simulink model "modules_intentions"  (R2017a)
settings: Solver=ode4  StartTime=0.0  StopTime=time_stop  FixedStep=time_step  RelTol=1e-3
undefined symbols (not defined in the file or in its folder): beta, Delta_guidance, Delta_matrix, eta_initial, initial_desired_psi_vector, initial_desired_u_vector, initial_next_waypoint_indexes, initial_obstacle_ship_states, initial_obstacle_ship_states_dot, initial_reference_psi_vector, initial_reference_u_vector, initial_SBMPC_desired_psi_vector, initial_SBMPC_desired_u_vector, initial_SBMPC_next_waypoint_indexes, initial_SBMPC_obstacle_ship_states, initial_SBMPC_obstacle_ship_states_dot, initial_SBMPC_reference_psi_vector, initial_SBMPC_reference_u_vector, initial_SBMPC_x_d_psi_matrix, initial_SBMPC_x_d_u_matrix, initial_state, initial_x_d_psi_matrix, initial_x_d_u_matrix, K_sway, K_yaw, Kp_feedback_linearization, kp_heading, Nmax, nu_initial, num_obs_ship_waypoints, num_prediction_time_steps, number_of_control_behaviors, number_of_obstacle_ships, number_of_SBMPC_obstacle_ships, obs_speed_between_waypoints, obstacle_waypoint_matrix, Omega_matrix, own_ship_reference_psi_init, own_ship_reference_speed, psi, Psi_init, radius_of_acceptance, SBMPC_obs_speed_between_waypoints, SBMPC_obstacle_waypoint_matrix, seconds_between_prediction, state_vector_init, T, T_k_surge, T_k_sway, T_k_yaw, T_s, T_waypoints, time_step, tsamp, U, U_init, V_init, waypoints_obstacle_ships, waypoints_own_ship, Xmax ... (+1)
(part 3 of 6)

== system modules_intentions/SBMPC obstacle ships/SBMPC using intentions /SBMPC obstacles: own-ship trajectory prediction ==
  note: each row = time step in prediction horizion
      | each column = a different control scenario
  note: each row = time step in prediction horizion
      | each column = a different control scenario
  note: each row = time step in prediction horizion
      | each column = a different control scenario
  note: each row = time step in prediction horizion
      | each column = a different control scenario
  note: each row = time step in prediction horizion
      | each column = a different control scenario
  t_0 : Inport
  SBMPC_obs_waypoints_matrix : Inport  Port=2
  "SBMPC_obs_eta_initial " : Inport  Port=3
  SBMPC_obs_nu_initial : Inport  Port=4
  SBMPC_obs_next_waypoint_index : Inport  Port=5
  Own ship trajectory prediction : MATLAB Function  TreatAsAtomicUnit=on
  To Workspace1 : ToWorkspace  Commented=on  VariableName=SBMPC_own_ship_x_predicted  SaveFormat=Structure With Time  SampleTime=tsamp
  To Workspace3 : ToWorkspace  Commented=on  VariableName=SBMPC_own_ship_y_predicted  SaveFormat=Structure With Time  SampleTime=tsamp
  To Workspace4 : ToWorkspace  Commented=on  VariableName=SBMPC_own_ship_heading_predicted  SaveFormat=Structure With Time  SampleTime=tsamp
  To Workspace5 : ToWorkspace  Commented=on  VariableName=SBMPC_own_ship_u_predicted  SaveFormat=Structure With Time  SampleTime=tsamp
  To Workspace6 : ToWorkspace  Commented=on  VariableName=SBMPC_own_ship_v_predicted  SaveFormat=Structure With Time  SampleTime=tsamp
  SBMPC_obs_own_ship_x_predicted : Outport  SampleTime=time_step
  SBMPC_obs_own_ship_y_predicted : Outport  Port=2  SampleTime=time_step
  SBMPC_obs_own_ship_heading_predicted : Outport  Port=3  SampleTime=time_step
  SBMPC_obs_own_ship_u_predicted : Outport  Port=4  SampleTime=time_step
  "SBMPC_obs_own_ship_v_predicted " : Outport  Port=5  SampleTime=time_step
  wires:
  SBMPC_obs_waypoints_matrix/1 -> Own ship trajectory prediction/4(waypoints_matrix)
  SBMPC_obs_nu_initial/1 -> Own ship trajectory prediction/3(nu_initial)
  "SBMPC_obs_eta_initial "/1 -> Own ship trajectory prediction/2(eta_initial)
  SBMPC_obs_next_waypoint_index/1 -> Own ship trajectory prediction/5(next_waypoint_index)
  t_0/1 -> Own ship trajectory prediction/1(t_0)
  Own ship trajectory prediction/1(own_ship_x_predicted) -> SBMPC_obs_own_ship_x_predicted/1, To Workspace1/1
  Own ship trajectory prediction/2(own_ship_y_predicted) -> SBMPC_obs_own_ship_y_predicted/1, To Workspace3/1
  Own ship trajectory prediction/3(own_ship_heading_predicted) -> To Workspace4/1, SBMPC_obs_own_ship_heading_predicted/1
  Own ship trajectory prediction/4(own_ship_u_predicted) -> SBMPC_obs_own_ship_u_predicted/1, To Workspace5/1
  Own ship trajectory prediction/5(own_ship_v_predicted) -> "SBMPC_obs_own_ship_v_predicted "/1, To Workspace6/1

== matlab function modules_intentions/Own-ship/Own-ship PSV/PSV/PSV model ==
  data: Pr input; psi_ca input; desired_nu input; state output; desired_psi input; time_step parameter; eta_initial parameter; nu_initial parameter; tau output; Kp_feedback_linearization parameter; kp_heading parameter; Xmax parameter; Ymax parameter; Nmax parameter; K_sway parameter; K_yaw parameter; T_k_surge parameter; T_k_sway parameter; T_k_yaw parameter
function [state, tau]   = PSV(Pr, psi_ca, desired_nu, desired_psi, time_step, eta_initial, nu_initial, Kp_feedback_linearization, kp_heading, Xmax, Ymax, Nmax, K_sway, K_yaw, T_k_surge, T_k_sway, T_k_yaw)  
    desired_u = desired_nu(1);
    desired_v = desired_nu(2);
    desired_r = desired_nu(3);

    persistent psv_vessel; %Persistent variables are local to the function in which they are declared, yet their values are retained in memory between calls to the function.
    
    if (isempty(psv_vessel))
        psvParameters = coder.load('PSVparameters');
        psvModelParameters = psvParameters.model_config;
        psv_vessel = PSVvessel_class(psvModelParameters, eta_initial, nu_initial, time_step, desired_psi, desired_nu, Kp_feedback_linearization, kp_heading, Xmax, Ymax, Nmax, K_sway, K_yaw, T_k_surge, T_k_sway, T_k_yaw);
    end
    
    desired_psi = desired_psi + psi_ca;
    desired_nu(1) = desired_nu(1)*Pr;

    
    [psv_vessel, tau] = psv_vessel.update_states(desired_psi, desired_nu);           
    state = psv_vessel.state;   
end

== matlab function modules_intentions/Own-ship/reference model psi/own ship reference model psi ==
  data: reference_psi input; x_d_new output; Omega_matrix parameter; time_step parameter; eta_initial parameter
function x_d_new = ownShipReferenceModelPsi(reference_psi, Omega_matrix, time_step, eta_initial)

persistent x_d %%[eta; eat_dot; eta_dotdot] = [x,y,psi, x_dot, y_dot, psi_dot, x_ddot, y_ddot, psi_ddot]

if isempty(x_d)
    x_d = [eta_initial(1);eta_initial(2);eta_initial(3);0;0;0;0;0;0];
end

x_d = referenceModelPsi(x_d, reference_psi, Omega_matrix, time_step);
x_d_new = x_d;
end

== matlab function modules_intentions/Own-ship/SBMPC USING INTENTIONS /Calculate control behaviors/Compute hazard ==
  settings: updateMethod=DISCRETE  sampleTime=time_step
  data: obstacle_ships_u input size=[num_prediction_time_steps, total_number_of_obstacle_ships]; obstacle_ships_v input size=[num_prediction_time_steps, total_number_of_obstacle_ships]; obstacle_ships_psi input size=[num_prediction_time_steps, total_number_of_obstacle_ships]; t_0 input; own_ship_x_predicted input size=[num_prediction_time_steps, number_of_control_behaviors]; own_ship_y_predicted input size=[num_prediction_time_steps, number_of_control_behaviors]; own_ship_u_predicted input size=[num_prediction_time_steps, number_of_control_behaviors]; own_ship_v_predicted input size=[num_prediction_time_steps, number_of_control_behaviors]; own_ship_heading_predicted input size=[num_prediction_time_steps, number_of_control_behaviors]; CLOSE output size=[number_of_control_behaviors, total_number_of_obstacle_ships, num_prediction_time_steps]; d_0 output size=[number_of_control_behaviors, total_number_of_obstacle_ships, num_prediction_time_steps]; obstacle_ships_x_predicted input size=[num_prediction_time_steps, total_number_of_obstacle_ships]; obstacle_ships_y_predicted input size=[num_prediction_time_steps, total_number_of_obstacle_ships]; OVERTAKEN output size=[number_of_control_behaviors, total_number_of_obstacle_ships, num_prediction_time_steps]; STARBOARD output size=[number_of_control_behaviors, total_number_of_obstacle_ships, num_prediction_time_steps]; chosen_HEAD_ON_out output; CROSSED output size=[number_of_control_behaviors, total_number_of_obstacle_ships, num_prediction_time_steps]; mu output size=[number_of_control_behaviors, total_number_of_obstacle_ships, num_prediction_time_steps]; num_prediction_time_steps parameter; heading_angle_offset_commands parameter; propulsion_commands parameter; total_number_of_obstacle_ships parameter; seconds_between_prediction parameter; d_cl parameter; phi_head_on parameter; phi_crossed parameter; phi_overtaken parameter; phi_ahead parameter; K_coll parameter; C output size=number_of_control_behaviors, total_number_of_obstacle_ships, num_prediction_time_steps; R output size=number_of_control_behaviors, total_number_of_obstacle_ships, num_prediction_time_steps; q parameter; p parameter; d_safe parameter; k_boundary parameter; k_circle parameter; k_Pr parameter; k_psi_port parameter; k_psi_starboard parameter; Delta_Pr parameter; vessel_length parameter; circle_obstacle_parameters parameter; boundary_obstacles_parameters parameter; k_Delta_psi_port parameter; k_Delta_psi_starboard parameter; kappa parameter; f output size=[1,number_of_control_behaviors]; g output size=[1,number_of_control_behaviors]; hazard output size=[1,number_of_control_behaviors]; rad2deg parameter; num_boundary_obstacles parameter; num_circle_obstacles parameter; chosen_C_out output; chosen_P_out output; chosen_FC_out output; chosen_R_out output; chosen_scaled_mu_out output; T_s parameter; chosen_Pr_out output; chosen_psi_ca_out output; C_worst output; R_worst output; scaled_mu_worst output; Pr_worst output; psi_ca_worst output; f_worst_out output; g_worst_out output; smallest_hazard_out output; largest_hazard_out output; f_out output; g_out output; r parameter; R_vector_out output size=[number_of_control_behaviors, total_number_of_obstacle_ships, num_prediction_time_steps]; circle_safety_margin parameter; p_boundary parameter; p_circle parameter; q_circle parameter; q_boundary parameter; boundary_margin parameter; k_role parameter; L_role parameter; ROLE_realtive_to_own_ship_module parameter; L_FC parameter; k_FC parameter; number_of_control_behaviors parameter; HEAD_ON_realtive_to_own_ship_module parameter; chosen_scenario_index_out output; t_detect_out output size=[1, total_number_of_obstacle_ships]; changing_obs parameter; number_of_obstacle_ships parameter; L_C parameter
 function [CLOSE, d_0, OVERTAKEN, STARBOARD, chosen_HEAD_ON_out, CROSSED,mu, C, R, f, g, hazard, chosen_C_out, chosen_P_out, chosen_FC_out, chosen_R_out, chosen_scaled_mu_out, chosen_Pr_out, chosen_psi_ca_out, C_worst, R_worst, scaled_mu_worst, Pr_worst, psi_ca_worst, f_worst_out, g_worst_out, smallest_hazard_out, largest_hazard_out, f_out, g_out, R_vector_out, chosen_scenario_index_out, t_detect_out]                         = computeTotalHazard(obstacle_ships_u, obstacle_ships_v, obstacle_ships_psi, t_0,own_ship_x_predicted, own_ship_y_predicted,own_ship_u_predicted,own_ship_v_predicted, own_ship_heading_predicted, obstacle_ships_x_predicted, obstacle_ships_y_predicted, num_prediction_time_steps, heading_angle_offset_commands, propulsion_commands, total_number_of_obstacle_ships, seconds_between_prediction, d_cl,phi_head_on, phi_crossed, phi_overtaken,phi_ahead,K_coll, q, p, d_safe,k_boundary, k_circle, k_Pr, k_psi_port, k_psi_starboard, Delta_Pr, vessel_length, circle_obstacle_parameters, boundary_obstacles_parameters, k_Delta_psi_port, k_Delta_psi_starboard,kappa, rad2deg, num_boundary_obstacles, num_circle_obstacles, T_s, r,  circle_safety_margin, p_boundary, p_circle, q_circle, q_boundary, boundary_margin, k_role, L_role, ROLE_realtive_to_own_ship_module, L_FC, k_FC, number_of_control_behaviors, HEAD_ON_realtive_to_own_ship_module, changing_obs, number_of_obstacle_ships, L_C)
    persistent chosen_C;
    persistent chosen_scenario_index;
    persistent chosen_R;
    persistent chosen_scaled_mu;
    persistent chosen_P_role;
    persistent chosen_FC;
    persistent chosen_HEAD_ON;
    persistent chosen_Pr;
    persistent chosen_psi_ca;
    persistent chosen_Pr_worst;
    persistent chosen_psi_ca_worst;
    persistent f_worst;
    persistent g_worst;
    persistent f_chosen;
    persistent g_chosen;
    persistent smallest_hazard;
    persistent largest_hazard;
    persistent scenario_index_with_min_hazard;
    persistent scenario_index_with_max_hazard;
    persistent t_detect;
    persistent t_detect_update;
    
    if (isempty(chosen_C))
        chosen_C = zeros(1,number_of_control_behaviors);%chosen_C_init;
        chosen_scenario_index = 0;
        chosen_R = zeros(1,number_of_control_behaviors);%chosen_R_init;
        chosen_scaled_mu = zeros(1,number_of_control_behaviors);%chosen_scaled_mu_init; 
        chosen_P_role = zeros(1,number_of_control_behaviors);%chosen_P_role_init;
        chosen_FC     = zeros(1,number_of_control_behaviors);
        chosen_HEAD_ON = zeros(1,number_of_control_behaviors);
        chosen_Pr = 1;
        chosen_psi_ca = 0;
        chosen_Pr_worst = 0;
        chosen_psi_ca_worst = 0;
        f_worst = 0;
        g_worst = 0;
        f_chosen = 0;
        g_chosen = 0;
        smallest_hazard = 0;
        largest_hazard = 0;
        scenario_index_with_min_hazard = -1;
        scenario_index_with_max_hazard = -1;
        t_detect = ones(1, total_number_of_obstacle_ships)*(-1);
        t_detect_update = ones(1, total_number_of_obstacle_ships);
        
    end

    CLOSE     = zeros(number_of_control_behaviors, total_number_of_obstacle_ships, num_prediction_time_steps);%CLOSE_init;         %3D matrix, 1. dim: scenario, 2. dim: obstacle, 3. dim: prediction horizon time step.
    OVERTAKEN = zeros(number_of_control_behaviors, total_number_of_obstacle_ships, num_prediction_time_steps);%OVERTAKEN_init; %3D matrix, 1. dim: scenario, 2. dim: obstacle, 3. dim: prediction horizon time step.
    STARBOARD = zeros(number_of_control_behaviors, total_number_of_obstacle_ships, num_prediction_time_steps);%STARBOARD_init; %3D matrix, 1. dim: scenario, 2. dim: obstacle, 3. dim: prediction horizon time step.
    HEAD_ON   = zeros(number_of_control_behaviors, total_number_of_obstacle_ships, num_prediction_time_steps);%HEAD_ON_init;     %3D matrix, 1. dim: scenario, 2. dim: obstacle, 3. dim: prediction horizon time step.
    CROSSED   = zeros(number_of_control_behaviors, total_number_of_obstacle_ships, num_prediction_time_steps);%CROSSED_init;     %3D matrix, 1. dim: scenario, 2. dim: obstacle, 3. dim: prediction horizon time step.
    mu        = zeros(number_of_control_behaviors, total_number_of_obstacle_ships, num_prediction_time_steps);%mu_init;               %3D matrix, 1. dim: scenario, 2. dim: obstacle, 3. dim: prediction horizon time step.
    scaled_mu = zeros(number_of_control_behaviors, total_number_of_obstacle_ships, num_prediction_time_steps);%scaled_mu_init; %3D matrix, 1. dim: scenario, 2. dim: obstacle, 3. dim: prediction horizon time step.
    d_0       = zeros(number_of_control_behaviors, total_number_of_obstacle_ships, num_prediction_time_steps);%d_0_init;             %3D matrix. distance between own ship and obstacle ship i at time t in scenario k. 1. dim: scenario, 2. dim: obstacle, 3. dim: prediction horizon time step
    f         = zeros(1,number_of_control_behaviors);%f_init;                 %vector.
    g         = zeros(1,number_of_control_behaviors);%g_init;                 %vector
    
    
    if (num_circle_obstacles > 0)
        g_circle_init  = zeros(number_of_control_behaviors, num_circle_obstacles, num_prediction_time_steps);
    else
        g_circle_init = 0;
    end    
    if (num_boundary_obstacles > 0)
        g_boundary_init = zeros(number_of_control_behaviors, num_boundary_obstacles, num_prediction_time_steps);
    else
        g_boundary_init = 0;
    end 
    g_circle  = g_circle_init;       %3D matrix. 1. dim = scneario, 2. dim = circle obstacle index, 3. dim = prediction horizon time step.
    g_boundary = g_boundary_init;   %3D matrix. 1. dim = scneario, 2. dim = circle obstacle index, 3. dim = prediction horizon time step.
    C = zeros(number_of_control_behaviors, total_number_of_obstacle_ships, num_prediction_time_steps);%C_init; %cost of collision. 3D matrix, 1. dim: scenario, 2. dim: obstacle, 3. dim: prediction horizon time step.
    R = zeros(number_of_control_behaviors, total_number_of_obstacle_ships, num_prediction_time_steps);%R_init; %Risk of collision. 3D matrix, 1. dim: scenario, 2. dim: obstacle, 3. dim: prediction horizon time step.
    hazard = zeros(1,number_of_control_behaviors);%hazard_init;
    P_role = zeros(number_of_control_behaviors, total_number_of_obstacle_ships, num_prediction_time_steps);%P_role_init;
    FC = zeros(number_of_control_behaviors, total_number_of_obstacle_ships, num_prediction_time_steps);%FC_init;
    
     
    Pr_last = chosen_Pr;     %the Pr corresponding to the previously calculated lowest hazard.
    psi_ca_last = chosen_psi_ca;    
    if (t_0 == 0)
        Pr_last = 1;
        psi_ca_last = 0;
    end
    
    if (mod(t_0, seconds_between_prediction) == 0) %only compute every "seconds_between_prediction" second.
        scenario_index = 0;
        for Pr = propulsion_commands
            for psi_ca = heading_angle_offset_commands 
                scenario_index = scenario_index + 1;                      
                prediction_time = 0;
                for t=1:num_prediction_time_steps   
                    prediction_time = t_0 + t*T_s;

                    %%%% Penalty for static obstacles   
                    if (num_circle_obstacles > 0)
                        circle_obs_counter = 0;
                        for circle_obstacle = circle_obstacle_parameters.'         %in each iteration, circle_obstacle is column vector with [radius; center_x; center_y]
                            circle_obs_counter = circle_obs_counter + 1;
                            radius    = circle_obstacle(1);
                            center_x  = circle_obstacle(2);
                            center_y  = circle_obstacle(3);
                            crossing_with_circle = SBMPC_isCollisionWithCircleObstacle(own_ship_x_predicted(t,scenario_index), own_ship_y_predicted(t,scenario_index), vessel_length, own_ship_heading_predicted(t,scenario_index), center_x, center_y, radius, circle_safety_margin);                       
                            vessel_bow_x = own_ship_x_predicted(t,scenario_index) + cos(own_ship_heading_predicted(t,scenario_index))*(vessel_length/2);
                            vessel_bow_y = own_ship_y_predicted(t,scenario_index) + sin(own_ship_heading_predicted(t,scenario_index))*(vessel_length/2);
                            distance_bow_to_circle_center = sqrt( (center_x - vessel_bow_x)^2 + (center_y - vessel_bow_y)^2 );
                            g_circle(scenario_index, circle_obs_counter, t) = (crossing_with_circle+1)*k_circle*(1/(prediction_time - t_0)^p_circle)*((radius+L_C)/ distance_bow_to_circle_center)^q_circle;%*(psi_ca*rad2deg)     * (1/distance_bow_to_circle_center)                   
                       end % end for
                    end % end if                        

                    if (num_boundary_obstacles > 0)
                        boundary_obs_counter = 0;
                        for boundary_obstacle = boundary_obstacles_parameters.'
                            boundary_obs_counter = boundary_obs_counter + 1;
                            boundary_start_x = boundary_obstacle(1);
                            boundary_start_y = boundary_obstacle(2);
                            boundary_end_x   = boundary_obstacle(3);
                            boundary_end_y   = boundary_obstacle(4);  
                            vessel_bow_x = own_ship_x_predicted(t,scenario_index) + cos(own_ship_heading_predicted(t,scenario_index))*(vessel_length/2);
                            vessel_bow_y = own_ship_y_predicted(t,scenario_index) + sin(own_ship_heading_predicted(t,scenario_index))*(vessel_length/2);
                            distance_bow_to_line = dist_from_bow_to_line( vessel_bow_x, vessel_bow_y, boundary_start_x, boundary_start_y, boundary_end_x, boundary_end_y ); % from http://paulbourke.net/geometry/pointlineplane/
                            crossing_with_boundary = SBMPC_isCollisionWithBoundaryObstacle(own_ship_x_predicted(t,scenario_index), own_ship_y_predicted(t,scenario_index), vessel_length, own_ship_heading_predicted(t,scenario_index), boundary_start_x, boundary_start_y, boundary_end_x, boundary_end_y);
                            g_boundary(scenario_index, boundary_obs_counter, t) = (crossing_with_boundary+1)*k_boundary*( 1 / (prediction_time - t_0)^p_boundary )*((boundary_margin)/(distance_bow_to_line))^q_boundary;  %from wiki https://en.wikipedia.org/wiki/Distance_from_a_point_to_a_line
                        end % end for
                    end % end if

                    for obstacle_ship_index = 1:total_number_of_obstacle_ships
                        obstacle_ship_speed = sqrt(obstacle_ships_u(t,obstacle_ship_index)^2 + obstacle_ships_v(t,obstacle_ship_index)^2);
                        own_ship_speed = sqrt(own_ship_u_predicted(t,scenario_index)^2 + own_ship_v_predicted(t,scenario_index)^2);
                        own_ship_u_NED = own_ship_speed*cos(own_ship_heading_predicted(t,scenario_index));
                        own_ship_v_NED = own_ship_speed*sin(own_ship_heading_predicted(t,scenario_index));
                        obstacle_ship_u_NED = obstacle_ship_speed*cos(obstacle_ships_psi(t,obstacle_ship_index));  
                        obstacle_ship_v_NED = obstacle_ship_speed*sin(obstacle_ships_psi(t,obstacle_ship_index));               
                        V_0 = [own_ship_u_NED,own_ship_v_NED];
                        V_i = [obstacle_ship_u_NED, obstacle_ship_v_NED];       
                                                
                        d_0(scenario_index, obstacle_ship_index, t) = sqrt((own_ship_x_predicted(t,scenario_index) - obstacle_ships_x_predicted(t,obstacle_ship_index))^2 ...
                                                                        +  (own_ship_y_predicted(t,scenario_index) - obstacle_ships_y_predicted(t,obstacle_ship_index))^2); 
                                                                    
                        if ( obstacle_ship_index <= number_of_obstacle_ships)   
                            if (changing_obs(obstacle_ship_index) == 1) %if it is a normal obs ship AND this normal obs ship is changing her waypoints midway in scenario
                                t_detect(obstacle_ship_index) = 1;
                                t_detect_update(obstacle_ship_index) = false;
                            elseif(changing_obs(obstacle_ship_index) == 0 && d_0(scenario_index, obstacle_ship_index, t) <= d_safe(obstacle_ship_index) && t_detect_update(obstacle_ship_index) == true)
                                t_detect(obstacle_ship_index) = t_0;
                                t_detect_update(obstacle_ship_index) = false;
                            end
                        elseif(obstacle_ship_index >number_of_obstacle_ships ) 
                            if (d_0(scenario_index, obstacle_ship_index, t) <= d_safe(obstacle_ship_index) && t_detect_update(obstacle_ship_index) == true)
                                t_detect(obstacle_ship_index) = t_0;
                                t_detect_update(obstacle_ship_index) = false;    
                            end
                        end
                                                                    
                        %%%% CLOSE
                                                                    
                        if (d_0(scenario_index, obstacle_ship_index, t) <= d_cl(obstacle_ship_index))
                            CLOSE(scenario_index, obstacle_ship_index, t) = 1;
                        else
                            CLOSE(scenario_index, obstacle_ship_index, t) = 0;
                        end % end if

                        %%%% OVERTAKEN                  
                        %equation 5 in johansen
                        epsilon = 1;
                        if (CLOSE(scenario_index, obstacle_ship_index, t) == 1 && obstacle_ship_speed > own_ship_speed + epsilon && dot(V_0, V_i) > cos(phi_overtaken)*norm(V_0)*norm(V_i))
                            OVERTAKEN(scenario_index, obstacle_ship_index, t) = 1;
                        else
                            OVERTAKEN(scenario_index, obstacle_ship_index, t) = 0;
                        end % end if

                        %%%% STARBOARD
                        L = [ obstacle_ships_x_predicted(t,obstacle_ship_index) - own_ship_x_predicted(t,scenario_index) , obstacle_ships_y_predicted(t,obstacle_ship_index) - own_ship_y_predicted(t,scenario_index) ];
                        L_unit_vector = L/norm(L);
                        L_angle = atan2(  (obstacle_ships_y_predicted(t,obstacle_ship_index) - own_ship_y_predicted(t,scenario_index)) , (obstacle_ships_x_predicted(t,obstacle_ship_index) - own_ship_x_predicted(t,scenario_index))  );

                        if (L_angle > own_ship_heading_predicted(t,scenario_index))
                            STARBOARD(scenario_index, obstacle_ship_index, t) = 1;
                        else
                            STARBOARD(scenario_index, obstacle_ship_index, t) = 0;
                        end
                        %rad2deg = 180/pi;
                        %L_angle_deg = L_angle*rad2deg;
                        %L_angle_deg_converted_to_positive =  mod((L_angle_deg + 360), 360);
                        %L_angle_mapped = L_angle_deg_converted_to_positive*deg2rad;  %map negative angles to positive angles.

                        %%%% HEAD_ON
                        head_on_condition = false;
                        if ( dot(V_0, V_i) < -cos(phi_head_on)*norm(V_0)*norm(V_i) && dot(V_0, L_unit_vector) > cos(phi_ahead)*norm(V_0) ) 
                            head_on_condition = true ; %equation 6-7 in johansen paper 
                        end% end if

                        if (CLOSE(scenario_index, obstacle_ship_index, t) == 1 && norm(V_i) ~= 0 && head_on_condition == true )
                            HEAD_ON(scenario_index, obstacle_ship_index, t) = 1;
                        else
                            HEAD_ON(scenario_index, obstacle_ship_index, t) = 0;
                        end % end if

                        %%%% CROSSED                                              
                        if (CLOSE(scenario_index, obstacle_ship_index, t) == 1 && dot(V_0, V_i) < cos(phi_crossed)*norm(V_0)*norm(V_i))
                            CROSSED(scenario_index, obstacle_ship_index, t) = 1;
                        else
                            CROSSED(scenario_index, obstacle_ship_index, t) = 0;
                        end % end if
                                                
                        %%%% RULE14    
                        if (CLOSE(scenario_index, obstacle_ship_index, t) == 1 && STARBOARD(scenario_index, obstacle_ship_index, t) == 1 && HEAD_ON(scenario_index, obstacle_ship_index, t) == 1 )
                            RULE14 = true;
                        else
                            RULE14 = false;
                        end % end if

                        %%%% RULE15   
                        if (CLOSE(scenario_index, obstacle_ship_index, t) == 1 && STARBOARD(scenario_index, obstacle_ship_index, t) == 1 && CROSSED(scenario_index, obstacle_ship_index, t) == 1 && OVERTAKEN(scenario_index, obstacle_ship_index, t)== 0 )
                            RULE15 = true;
                        else
                             RULE15 = false;
                        end % end if

                        %%%% mu
                        if (RULE14 || RULE15)
                            mu(scenario_index, obstacle_ship_index, t) =  1;
                        else
                            mu(scenario_index, obstacle_ship_index, t) = 0;
                        end % end if                         
                        scaled_mu(scenario_index, obstacle_ship_index, t) = kappa(obstacle_ship_index)*mu(scenario_index, obstacle_ship_index, t);
                        
                        
                        %%%% Role variable 
                        if (CLOSE(scenario_index, obstacle_ship_index, t) == 1 && d_0(scenario_index, obstacle_ship_index, t) >= L_role)
                            HEAD_ON_intention_value = HEAD_ON_realtive_to_own_ship_module(obstacle_ship_index);
                            P_role(scenario_index, obstacle_ship_index, t) = ROLE_realtive_to_own_ship_module(obstacle_ship_index)*k_role*(1-HEAD_ON_intention_value)*(sqrt(abs(psi_ca*rad2deg)) + 1 - Pr);        
                        else
                            P_role(scenario_index, obstacle_ship_index, t) = 0;
                        end % end if
                        
                        
                                                                 
                        %%%% Cost of collision
                        C(scenario_index, obstacle_ship_index, t) = K_coll(obstacle_ship_index)*norm(V_0 - V_i)^2;
                        
                        %%%% Risk of collision    
                        
                        if (d_0(scenario_index, obstacle_ship_index, t) <= L_FC)
                            FC(scenario_index, obstacle_ship_index, t) = 1;
                        else
                            FC(scenario_index, obstacle_ship_index, t) = 0;
                        end % end if
                        
                        
                        if (d_0(scenario_index, obstacle_ship_index, t) <= d_safe(obstacle_ship_index) && d_0(scenario_index, obstacle_ship_index, t) >= 20)                          
                            R(scenario_index, obstacle_ship_index, t)  = (1 / (abs(prediction_time - t_0)^p))*( r*( d_safe(obstacle_ship_index) / d_0(scenario_index, obstacle_ship_index, t) )^q  + k_FC*FC(scenario_index, obstacle_ship_index, t)   ) ;
                            if ( R(scenario_index, obstacle_ship_index, t) >= 20000)
                                R(scenario_index, obstacle_ship_index, t) = 20000;  %saturate
                            end
                        else
                            R(scenario_index, obstacle_ship_index, t) = 0;
                        end % end if        
                        
                    end % end for - num obs ships            
                end % end for - time steps                                        
            end % end for - psi_ca
        end % end for - Pr     
        
        scenario_index = 0;
        for Pr = propulsion_commands
            for psi_ca = heading_angle_offset_commands 
                scenario_index = scenario_index + 1;
                sum_matrix = C(scenario_index,:,:).*R(scenario_index,:,:) + scaled_mu(scenario_index,:,:) + P_role(scenario_index,:,:);   %sum matrix: 1. dim = control behavior, 2. dim = obstacle, 3. dim = prediction horizon time step.
                %assert (size(sum_matrix) == [1, total_number_of_obstacle_ships, num_prediction_time_steps]);
                sum_matrix = reshape(sum_matrix, total_number_of_obstacle_ships, num_prediction_time_steps);
                [best_value,idx] = max(sum_matrix(:));
                [best_obstacle_ship_index,best_timestep] = ind2sub(size(sum_matrix),idx);
                  
                  %ALTERNATIVE WAY TO FIND MAXIMUMS
%                 max_sum = -1;
%                 i_ = 0;
%                 t_ = 0;
%                 
%                 for i = 1:total_number_of_obstacle_ships
%                     for t = 1:num_prediction_time_steps
%                         sum = C(scenario_index, i, t)*R(scenario_index, i, t) + scaled_mu(scenario_index, i, t) + P_role(scenario_index, i, t);
%                         if (sum > max_sum)
%                             max_sum = sum;
%                             i_ = i;
%                             t_ = t;
%                         end % end if
%                     end % end for
%                 end % end for%                 
%                 assert (best_value == max_sum);                            
                
                if ( psi_ca < 0)
                    k_psi = k_psi_port;  
                    Delta_psi = k_Delta_psi_port*(abs(psi_ca*rad2deg - psi_ca_last*rad2deg));
                else
                    k_psi = k_psi_starboard;
                    Delta_psi = k_Delta_psi_starboard*(abs(psi_ca*rad2deg - psi_ca_last*rad2deg));
                end % end if                
                
                f(scenario_index) = k_Pr*(1-Pr) + k_psi*(abs(psi_ca*rad2deg)) + Delta_Pr*abs(Pr - Pr_last) + Delta_psi ;                                 
                
                g_circle_scenario = 0;
                if (num_circle_obstacles > 0)
                    g_circle_scenario_values = g_circle(scenario_index, :, :);
                    g_circle_scenario = max(g_circle_scenario_values(:));
                end % end if                
                g_boundary_scenario = 0;
                if (num_boundary_obstacles > 0)
                    g_boundary_scenario_values = g_boundary(scenario_index, :, :);
                    g_boundary_scenario = max(g_boundary_scenario_values(:));
                end % end if                
                g(scenario_index) = g_circle_scenario + g_boundary_scenario;
                
                hazard(scenario_index) = best_value + f(scenario_index) + g(scenario_index);

                %The C, R and K*µ corresponding to the values used to find hazard H for scenario k.
                chosen_C(scenario_index) = C(scenario_index,best_obstacle_ship_index,best_timestep);  %the C value used to compute hazard in scenario number "scenario_index"
                chosen_R(scenario_index) = R(scenario_index,best_obstacle_ship_index,best_timestep);
                
                chosen_scaled_mu(scenario_index) = scaled_mu(scenario_index,best_obstacle_ship_index,best_timestep);  
                chosen_P_role(scenario_index) = P_role(scenario_index,best_obstacle_ship_index,best_timestep);
                chosen_FC(scenario_index)     = FC(scenario_index,best_obstacle_ship_index,best_timestep)*k_FC;
                
                chosen_HEAD_ON(scenario_index) = HEAD_ON(scenario_index, best_obstacle_ship_index, best_timestep);
                
                assert (best_value == chosen_C(scenario_index)*chosen_R(scenario_index) + chosen_scaled_mu(scenario_index) + chosen_P_role(scenario_index));                                           
            end % end for
        end % end for
        
        [min_hazard, scenario_index_with_min_hazard] = min(hazard);
        [max_hazard, scenario_index_with_max_hazard] = max(hazard);  
        smallest_hazard = min_hazard;
        largest_hazard = max_hazard;
        
        assert(min_hazard == hazard(scenario_index_with_min_hazard));
        assert(max_hazard == hazard(scenario_index_with_max_hazard));
        
        f_chosen = f(scenario_index_with_min_hazard);
        g_chosen = g(scenario_index_with_min_hazard);
        f_worst  = f(scenario_index_with_max_hazard);
        g_worst  = g(scenario_index_with_max_hazard); 
        
        
       
        scenario_index = 0;
        for Pr = propulsion_commands
            for psi_ca = heading_angle_offset_commands
                scenario_index = scenario_index +1;
                if (scenario_index == scenario_index_with_min_hazard)
                    chosen_Pr = Pr;
                    chosen_psi_ca = psi_ca;
                    chosen_scenario_index = scenario_index;
                elseif (scenario_index == scenario_index_with_max_hazard)
                    chosen_Pr_worst = Pr;
                    chosen_psi_ca_worst = psi_ca;                   
                end % end if
            end % end for
        end % end for                  
    end % end if
 
    chosen_C_out = chosen_C(scenario_index_with_min_hazard);
    chosen_scenario_index_out = chosen_scenario_index;
    chosen_P_out = chosen_P_role(scenario_index_with_min_hazard);
    chosen_FC_out = chosen_FC(scenario_index_with_min_hazard);
    chosen_HEAD_ON_out = chosen_HEAD_ON(scenario_index_with_min_hazard);
    C_worst = chosen_C(scenario_index_with_max_hazard);
    P_worst = chosen_P_role(scenario_index_with_max_hazard);
    chosen_R_out = chosen_R(scenario_index_with_min_hazard);
    R_worst = chosen_R(scenario_index_with_max_hazard);
    chosen_scaled_mu_out = chosen_scaled_mu(scenario_index_with_min_hazard);
    scaled_mu_worst = chosen_scaled_mu(scenario_index_with_max_hazard);
    chosen_Pr_out = chosen_Pr;
    Pr_worst = chosen_Pr_worst;
    chosen_psi_ca_out = chosen_psi_ca;
    psi_ca_worst = chosen_psi_ca_worst;
    f_worst_out = f_worst;
    g_worst_out = g_worst;
    R_vector_out = R;
    
    f_out = f_chosen;
    g_out = g_chosen;
    smallest_hazard_out = smallest_hazard;
    largest_hazard_out =  largest_hazard;
    
    t_detect_out = t_detect;
end

== matlab function modules_intentions/Own-ship/Own-ship PSV/derivative/vector derivative ==
  data: x input; derivative output; x_previous input; time_step parameter
function derivative = derivativeVector(x, x_previous, time_step)
derivative = [0;0;0];    
derivative(1) = (x(1) - x_previous(1))/time_step;
derivative(2) = (x(2) - x_previous(2))/time_step;
derivative(3) = (x(3) - x_previous(3))/time_step;
end
